simulink model "rlVarth"  (R2020b)
settings: Solver=ode23t  StartTime=0.0  StopTime=Tf  RelTol=1e-2
libraries: rllib x1
settings Model: Creator=The MathWorks, Inc.  LastModifiedBy=mluser

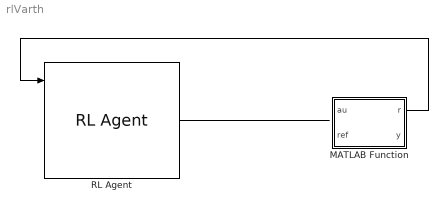
== system rlVarth ==
  MATLAB Function : MATLAB Function  TreatAsAtomicUnit=on
  RL Agent : rllib/RL Agent  Agent=agentObj  ProvideReward=on  ProvideIsDone=on  ProvideCumRwd=off  TreatAsDirectFeedthrough=on  CollectLoggedSignals=on  CollectModelStates=on
  wires:
  RL Agent/1 -> ?
  MATLAB Function/1(r) -> RL Agent/1

== matlab function rlVarth/MATLAB Function ==
  data: r output; au input; ref input; y output
function [r,y] = fcn(au,ref)
    A=2;B=2;K=1.5;C=1;
    r=x-ref;
    u=-K*r+au;
    x= A*x+B*u;
    y=C*x;
